simulink model "robertto1DOF"  (R2018a)
settings: Solver=VariableStepAuto  StartTime=0.0  StopTime=200  MaxStep=0.1  RelTol=1e-8
InitFcn:
  | RLDesignJoystick
  | 
  | load('joystick_ref_002.mat')
  | % global t_change;
  | % t_change=0;
  | 
  | % T = 20;
  | a = 0.5;
  | b = 1;
  | v0 = 1;
  | tau = 0.5;
  | %tau=10;
  | 
  | % PID Gains
  | kp = 0.5;
  | % kp = 2*b/a^2;
  | TI = 5;
  | TD = 0.1;
  | 
  | % SM Gains
  | k0 = 20;
  | k1 = 0.05;
  | 
  | % DAS
  | DT=4;
  | % gamma1sq=0.05;
  | % gamma2sq=0.3;
  | gamma1sq=0.025;
  | gamma2sq=0.01;
  | y_ref=0;
values from neighbouring files (symbols this model uses):
  a2 = 26.4940946148    [CrossTrackUSV.mat]
  b2 = 0.266666666667    [CrossTrackUSV.mat]
  K2 = 1619.40576956    [CrossTrackUSV.mat]
libraries: simulink x8, vrlib x1, realtime_pacer_lib x1
settings Model: Creator=KvonEllenrieder  LastModifiedBy=transmogrifier
settings SolverCC: ZeroCrossAlgorithm=Adaptive
settings DebuggingCC: IgnoredZcDiagnostic=none
settings CodeAppCC: StateflowObjectComments=on

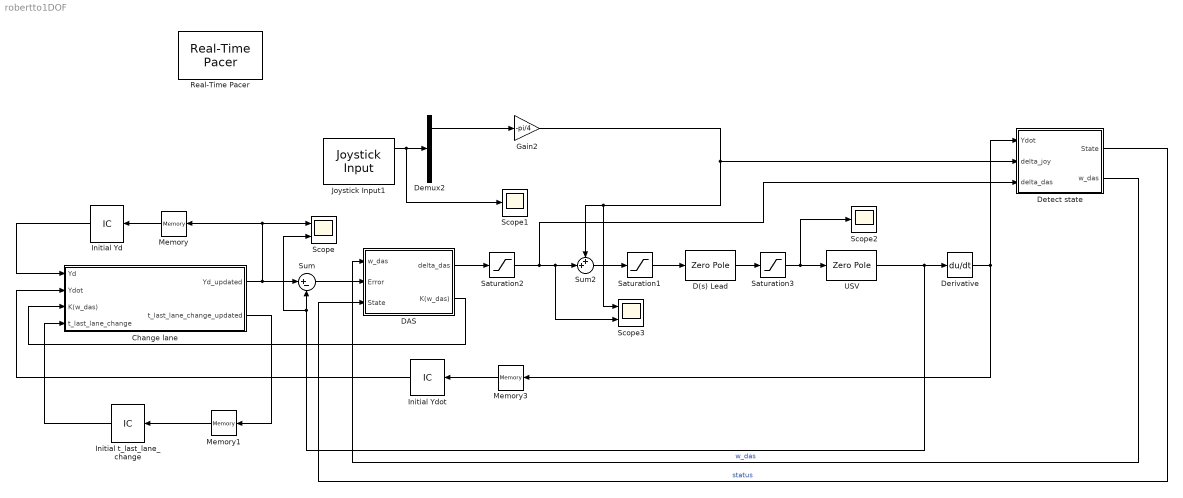
== system robertto1DOF ==
  Change lane : Subsystem
  D(s) Lead : ZeroPole  Zeros=[-b2]  Poles=[-a2]  Gain=[K2]
  DAS : Subsystem
  Demux2 : Demux  Outputs=8
  Derivative : Derivative
  Detect state : Subsystem
  Gain2 : Gain  Gain=-pi/4
  Initial Yd : InitialCondition  Value=0
  Initial Ydot : InitialCondition  Value=0
  Initial t_last_lane_change : InitialCondition  Value=0
  Joystick Input1 : vrlib/Joystick Input  joyid=1  adjustports=on  forcefeed=off
      settings: SourceProductBaseCode=VR
  Memory : Memory
  Memory1 : Memory
  Memory3 : Memory
  Real-Time Pacer : realtime_pacer_lib/Real-Time Pacer  simTimePerRealTime=1
  Saturation1 : Saturate  UpperLimit=pi/4  LowerLimit=-pi/4
  Saturation2 : Saturate  UpperLimit=pi/4  LowerLimit=-pi/4
  Saturation3 : Saturate  UpperLimit=pi/4  LowerLimit=-pi/4
  Scope : Scope  NumInputPorts=2
  Scope1 : Scope
  Scope2 : Scope
  Scope3 : Scope  NumInputPorts=2
  Sum : Sum  Inputs=|+-
  Sum2 : Sum  Inputs=++|
  USV : ZeroPole  Zeros=[]  Poles=[0 0 -3]  Gain=[2]
  wires:
  Change lane/1(Yd_updated) -> Memory/1, Scope/1, Sum/1
  Detect state/1(State) -> DAS/3(State)  "status"
  Joystick Input1/1 -> Scope1/1, Demux2/1
  Sum2/1 -> Saturation1/1
  Detect state/2(w_das) -> DAS/1(w_das)  "w_das"
  Gain2/1 -> Scope3/1, Sum2/1, Detect state/2(delta_joy)
  Sum/1 -> DAS/2(Error)
  Memory/1 -> Initial Yd/1
  Initial Yd/1 -> Change lane/1(Yd)
  Change lane/2(t_last_lane_change_updated) -> Memory1/1
  Memory1/1 -> Initial t_last_lane_change/1
  Initial t_last_lane_change/1 -> Change lane/4(t_last_lane_change)
  Saturation2/1 -> Detect state/3(delta_das), Scope3/2, Sum2/2
  DAS/2(K(w_das)) -> Change lane/3(K(w_das))
  DAS/1(delta_das) -> Saturation2/1
  Initial Ydot/1 -> Change lane/2(Ydot)
  Memory3/1 -> Initial Ydot/1
  Demux2/2 -> Gain2/1
  USV/1 -> Derivative/1, Scope/2, Sum/2
  D(s) Lead/1 -> Saturation3/1
  Derivative/1 -> Memory3/1, Detect state/1(Ydot)
  Saturation1/1 -> D(s) Lead/1
  Saturation3/1 -> USV/1, Scope2/1

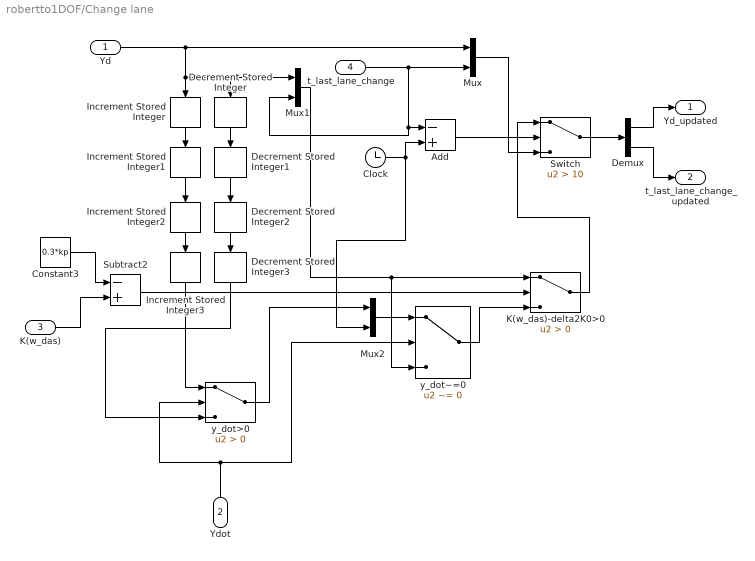
== system robertto1DOF/Change lane ==
  Yd : Inport
  Ydot : Inport  Port=2
  K(w_das) : Inport  Port=3
  t_last_lane_change : Inport  Port=4
  Add : Sum  Inputs=-+
  Clock : Clock
  Constant3 : Constant  Value=0.3*kp
  Decrement Stored Integer{,1..3} (4 alike) : simulink/Additional Math & Discrete/Additional Math: Increment - Decrement/Decrement Stored Integer
      settings: SourceProductName=Simulink  SourceProductBaseCode=SL
  Demux : Demux  Outputs=2
  Increment Stored Integer{,1..3} (4 alike) : simulink/Additional Math & Discrete/Additional Math: Increment - Decrement/Increment Stored Integer
      settings: SourceProductName=Simulink
  K(w_das)-delta2K0>0 : Switch  Criteria=u2 > Threshold  ZeroCross=off
  Mux : Mux  Inputs=2
  Mux1 : Mux  Inputs=2
  Mux2 : Mux  Inputs=2
  Subtract2 : Sum  Inputs=-+
  Switch : Switch  Criteria=u2 > Threshold  Threshold=10
  y_dot>0 : Switch  Criteria=u2 > Threshold
  y_dot~=0 : Switch  Criteria=u2 ~= 0
  Yd_updated : Outport
  t_last_lane_change_updated : Outport  Port=2
  wires:
  Increment Stored Integer/1 -> Increment Stored Integer1/1
  y_dot>0/1 -> Mux2/1
  K(w_das)/1 -> Subtract2/2
  Yd/1 -> Mux/1, Mux1/1, Decrement Stored Integer/1, Increment Stored Integer/1
  y_dot~=0/1 -> K(w_das)-delta2K0>0/3
  Constant3/1 -> Subtract2/1
  Ydot/1 -> y_dot~=0/2, y_dot>0/2
  Decrement Stored Integer/1 -> Decrement Stored Integer1/1
  Clock/1 -> Mux2/2, Add/2
  t_last_lane_change/1 -> Mux1/2, Add/1, Mux/2
  Add/1 -> Switch/2
  K(w_das)-delta2K0>0/1 -> Switch/1
  Mux/1 -> Switch/3
  Switch/1 -> Demux/1
  Demux/1 -> Yd_updated/1
  Demux/2 -> t_last_lane_change_updated/1
  Mux1/1 -> K(w_das)-delta2K0>0/1, y_dot~=0/3
  Mux2/1 -> y_dot~=0/1
  Subtract2/1 -> K(w_das)-delta2K0>0/2
  Increment Stored Integer1/1 -> Increment Stored Integer2/1
  Increment Stored Integer2/1 -> Increment Stored Integer3/1
  Increment Stored Integer3/1 -> y_dot>0/1
  Decrement Stored Integer1/1 -> Decrement Stored Integer2/1
  Decrement Stored Integer2/1 -> Decrement Stored Integer3/1
  Decrement Stored Integer3/1 -> y_dot>0/3

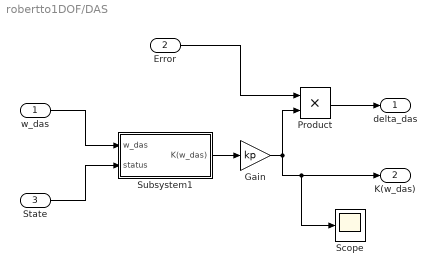
== system robertto1DOF/DAS ==
  w_das : Inport
  Error : Inport  Port=2
  State : Inport  Port=3
  Gain : Gain  Gain=kp
  Product : Product
  Scope : Scope
  Subsystem1 : Subsystem
  delta_das : Outport
  K(w_das) : Outport  Port=2
  wires:
  Product/1 -> delta_das/1
  Error/1 -> Product/1
  State/1 -> Subsystem1/2(status)
  Subsystem1/1(K(w_das)) -> Gain/1
  Gain/1 -> Product/2, Scope/1, K(w_das)/1
  w_das/1 -> Subsystem1/1(w_das)

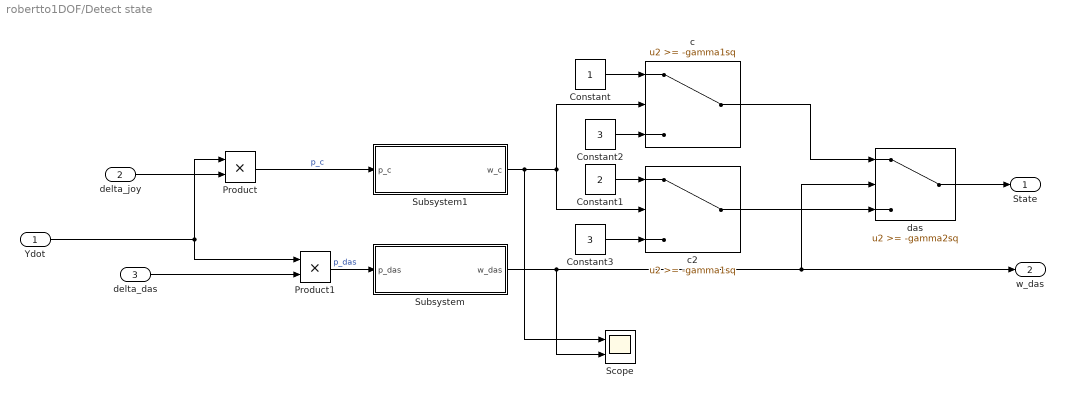
== system robertto1DOF/Detect state ==
  Ydot : Inport
  delta_joy : Inport  Port=2
  delta_das : Inport  Port=3
  Constant : Constant
  Constant1 : Constant  Value=2
  Constant2 : Constant  Value=3
  Constant3 : Constant  Value=3
  Product : Product
  Product1 : Product
  Scope : Scope  NumInputPorts=2
  Subsystem : Subsystem
  Subsystem1 : Subsystem
  c : Switch  Threshold=-gamma1sq
  c2 : Switch  Threshold=-gamma1sq
  das : Switch  Threshold=-gamma2sq
  State : Outport
  w_das : Outport  Port=2
  wires:
  Ydot/1 -> Product/1, Product1/1
  delta_joy/1 -> Product/2
  delta_das/1 -> Product1/2
  Product/1 -> Subsystem1/1(p_c)  "p_c"
  Product1/1 -> Subsystem/1(p_das)  "p_das"
  Subsystem/1(w_das) -> Scope/2, w_das/1, das/2
  Subsystem1/1(w_c) -> Scope/1, c2/2, c/2
  Constant/1 -> c/1
  c/1 -> das/1
  Constant1/1 -> c2/1
  c2/1 -> das/3
  Constant3/1 -> c2/3
  Constant2/1 -> c/3
  das/1 -> State/1

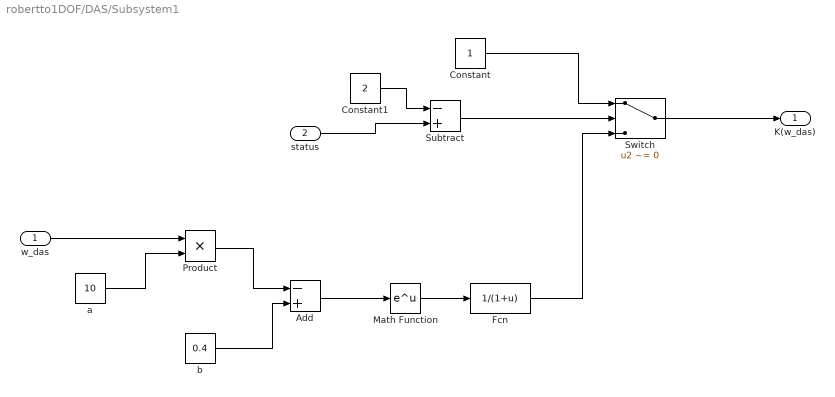
== system robertto1DOF/DAS/Subsystem1 ==
  w_das : Inport
  status : Inport  Port=2
  Add : Sum  Inputs=-+
  Constant : Constant
  Constant1 : Constant  Value=2
  Fcn : Fcn  Expr=1/(1+u)
  Math Function : Math  SaturateOnIntegerOverflow=on
  Product : Product
  Subtract : Sum  Inputs=-+
  Switch : Switch  Criteria=u2 ~= 0
  a : Constant  Value=10
  b : Constant  Value=0.4
  K(w_das) : Outport
  wires:
  w_das/1 -> Product/1
  a/1 -> Product/2
  Product/1 -> Add/1
  b/1 -> Add/2
  Add/1 -> Math Function/1
  Math Function/1 -> Fcn/1
  Fcn/1 -> Switch/3
  Constant/1 -> Switch/1
  Switch/1 -> K(w_das)/1
  Constant1/1 -> Subtract/1
  status/1 -> Subtract/2
  Subtract/1 -> Switch/2

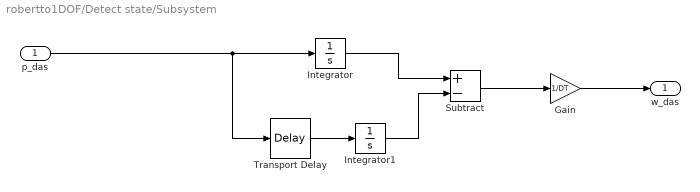
== system robertto1DOF/Detect state/Subsystem ==
  p_das : Inport
  Gain : Gain  Gain=1/DT
  Integrator : Integrator
  Integrator1 : Integrator
  Subtract : Sum  Inputs=+-
  Transport Delay : TransportDelay  DelayTime=DT
  w_das : Outport
  wires:
  Subtract/1 -> Gain/1
  Gain/1 -> w_das/1
  Transport Delay/1 -> Integrator1/1
  Integrator1/1 -> Subtract/2
  Integrator/1 -> Subtract/1
  p_das/1 -> Transport Delay/1, Integrator/1

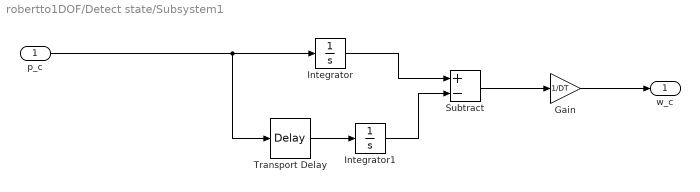
== system robertto1DOF/Detect state/Subsystem1 ==
  p_c : Inport
  Gain : Gain  Gain=1/DT
  Integrator : Integrator
  Integrator1 : Integrator
  Subtract : Sum  Inputs=+-
  Transport Delay : TransportDelay  DelayTime=DT
  w_c : Outport
  wires:
  p_c/1 -> Integrator/1, Transport Delay/1
  Integrator/1 -> Subtract/1
  Integrator1/1 -> Subtract/2
  Transport Delay/1 -> Integrator1/1
  Gain/1 -> w_c/1
  Subtract/1 -> Gain/1
